simulink model "PID_PD_LQR_Control_Quadrotor"  (R2012b)
settings: Solver=ode3  StartTime=0.0  StopTime=105  FixedStep=0.01  RelTol=1e-2
libraries: vrlib x2
settings Model: Creator=hellb  LastModifiedBy=hellb
settings OptimizationCC: ExpressionDepthLimit=128
settings DebuggingCC: UnderspecifiedInitializationDetection=Simplified  MergeDetectMultiDrivingBlocksExec=error  SolverPrmCheckMsg=none  FrameProcessingCompatibilityMsg=error  StateNameClashWarn=none
settings CodeAppCC: CustomSymbolStrType=$N$R$M_T
settings GRTTargetCC: CodeReplacementLibrary=C89/C90 (ANSI)

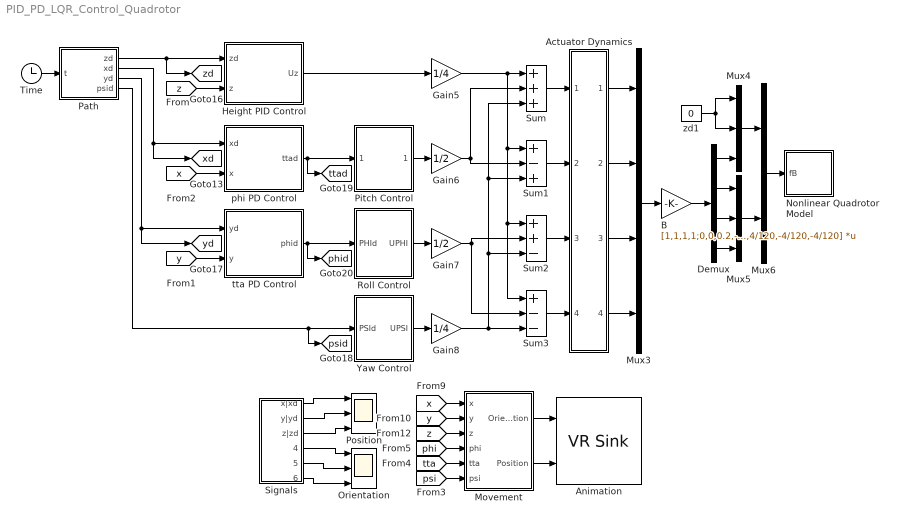
== system PID_PD_LQR_Control_Quadrotor ==
  Actuator Dynamics : Subsystem
  Animation : vrlib/VR Sink  InstantiateOnLoad=on  SampleTime=0.01  ViewEnable=on  RemoteChange=off  RemoteView=off  FieldsWritten=Drone.rotation.4.1.1.double#Drone.translation.3.1.1.double  WorldFileName=Animation\hummingbird.wrl  AutoView=off  VideoDimensions=[]  AllowVariableSize=off
  B : Gain  Gain=[1,1,1,1;0,0,0.2,-0.2;0.2,-0.2,0,0;4/120,4/120,-4/120,-4/120]  Multiplication=Matrix(K*u)
  Demux : Demux
  Gain5 : Gain  Gain=1/4
  Gain6 : Gain  Gain=1/2
  Gain7 : Gain  Gain=1/2
  Gain8 : Gain  Gain=1/4
  Height PID Control : Subsystem
  Movement : Subsystem
  Mux3 : Mux
  Mux4 : Mux  Inputs=3
  Mux5 : Mux  Inputs=3
  Mux6 : Mux  Inputs=2
  Nonlinear Quadrotor Model : Subsystem
  Orientation : Scope  NumInputPorts=3
      settings: YMin=-0.0225~-0.0075~-0.00015  YMax=0.0075~0.0225~0.00015  SaveName=Orientation
  Path : MATLAB Function  TreatAsAtomicUnit=on
      settings: PermitHierarchicalResolution=ParametersOnly
  Pitch Control : Subsystem
  Position : Scope  NumInputPorts=3
      settings: YMin=-0.25~-0.1~-0.25  YMax=3.25~1.3~3  SaveName=Position
  Roll Control : Subsystem
  Signals : Subsystem
  Sum : Sum  Inputs=+++
  Sum1 : Sum  Inputs=+-+
  Sum2 : Sum  Inputs=++-
  Sum3 : Sum  Inputs=+--
  Time : Clock
  Yaw Control : Subsystem
  phi PD Control : Subsystem
  tta PD Control : Subsystem
  zd1 : Constant  Value=0
  tag scope: phid=global, psid=global, ttad=global, xd=global, yd=global, zd=global
  wires:
  tta PD Control/1(phid) -> Roll Control/1(PHId), [phid]
  phi PD Control/1(ttad) -> Pitch Control/1(TTAd), [ttad]
  Height PID Control/1(Uz) -> Gain5/1
  Yaw Control/1(UPSI) -> Gain8/1
  Mux3/1 -> B/1
  B/1 -> Demux/1
  Demux/1 -> Mux4/3
  zd1/1 -> Mux4/1, Mux4/2
  Demux/2 -> Mux5/1
  Demux/3 -> Mux5/2
  Demux/4 -> Mux5/3
  Mux4/1 -> Mux6/1
  Mux5/1 -> Mux6/2
  [x] -> phi PD Control/2(x)
  Roll Control/1(UPHI) -> Gain7/1
  Pitch Control/1(UTTA) -> Gain6/1
  Gain5/1 -> Sum/1, Sum1/1, Sum3/1, Sum2/1
  [y] -> tta PD Control/2(y)
  Gain6/1 -> Sum1/2, Sum/2
  Gain7/1 -> Sum2/2, Sum3/2
  Gain8/1 -> Sum3/3, Sum2/3, Sum/3, Sum1/3
  [z] -> Height PID Control/2(z)
  Sum/1 -> Actuator Dynamics/1(U1)
  Sum1/1 -> Actuator Dynamics/2(U2)
  Sum2/1 -> Actuator Dynamics/3(U3)
  Sum3/1 -> Actuator Dynamics/4(U4)
  Actuator Dynamics/1(F1) -> Mux3/1
  Actuator Dynamics/2(F2) -> Mux3/2
  Actuator Dynamics/3(F3) -> Mux3/3
  Actuator Dynamics/4(F4) -> Mux3/4
  Mux6/1 -> Nonlinear Quadrotor Model/1(fB)
  Signals/1(x|xd) -> Position/1
  Signals/2(y|yd) -> Position/2
  Signals/3(z|zd) -> Position/3
  Signals/4(phi|phid) -> Orientation/1
  Signals/5(tta|ttad) -> Orientation/2
  Signals/6(psi|psid) -> Orientation/3
  Time/1 -> Path/1(t)
  Path/1(zd) -> [zd], Height PID Control/1(zd)
  Path/2(xd) -> phi PD Control/1(xd), [xd]
  Path/3(yd) -> tta PD Control/1(yd), [yd]
  Path/4(psid) -> Yaw Control/1(PSId), [psid]
  [phi] -> Movement/4(phi)
  [psi] -> Movement/6(psi)
  [tta] -> Movement/5(tta)
  [x] -> Movement/1(x)
  [z] -> Movement/3(z)
  [y] -> Movement/2(y)
  Movement/1(Orientation) -> Animation/1
  Movement/2(Position) -> Animation/2

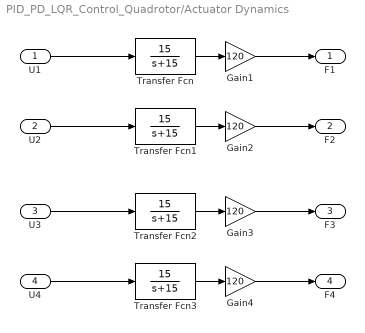
== system PID_PD_LQR_Control_Quadrotor/Actuator Dynamics ==
  U1 : Inport
  U2 : Inport  Port=2
  U3 : Inport  Port=3
  U4 : Inport  Port=4
  Gain{1..4} (4 alike) : Gain  Gain=120
  Transfer Fcn{,1..3} (4 alike) : TransferFcn  Numerator=[15]  Denominator=[1 15]
  F1 : Outport
  F2 : Outport  Port=2
  F3 : Outport  Port=3
  F4 : Outport  Port=4
  wires:
  Transfer Fcn1/1 -> Gain2/1
  U1/1 -> Transfer Fcn/1
  Gain2/1 -> F2/1
  Gain1/1 -> F1/1
  Transfer Fcn/1 -> Gain1/1
  Gain3/1 -> F3/1
  U3/1 -> Transfer Fcn2/1
  U4/1 -> Transfer Fcn3/1
  Transfer Fcn3/1 -> Gain4/1
  Gain4/1 -> F4/1
  U2/1 -> Transfer Fcn1/1
  Transfer Fcn2/1 -> Gain3/1

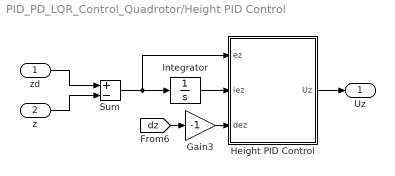
== system PID_PD_LQR_Control_Quadrotor/Height PID Control ==
  zd : Inport
  z : Inport  Port=2
  Gain3 : Gain  Gain=-1
  Height PID Control : MATLAB Function  TreatAsAtomicUnit=on
      settings: PermitHierarchicalResolution=ParametersOnly
  Integrator : Integrator
  Sum : Sum  Inputs=+-
  Uz : Outport
  wires:
  zd/1 -> Sum/1
  z/1 -> Sum/2
  Sum/1 -> Height PID Control/1(ez), Integrator/1
  Integrator/1 -> Height PID Control/2(iez)
  Gain3/1 -> Height PID Control/3(dez)
  [dz] -> Gain3/1
  Height PID Control/1(Uz) -> Uz/1

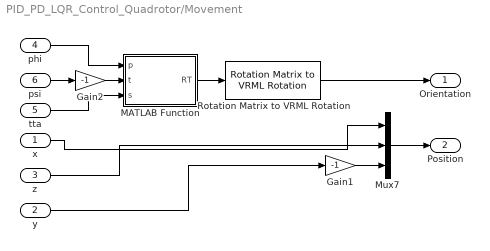
== system PID_PD_LQR_Control_Quadrotor/Movement ==
  x : Inport
  y : Inport  Port=2
  z : Inport  Port=3
  phi : Inport  Port=4
  tta : Inport  Port=5
  psi : Inport  Port=6
  Gain1 : Gain  Gain=-1
  Gain2 : Gain  Gain=-1
  MATLAB Function : MATLAB Function  TreatAsAtomicUnit=on
      settings: PermitHierarchicalResolution=ParametersOnly
  Mux7 : Mux  Inputs=3
  Rotation Matrix to VRML Rotation : vrlib/Utilities/Rotation Matrix to VRML Rotation  maxzero=1e-12
  Orientation : Outport
  Position : Outport  Port=2
  wires:
  Gain1/1 -> Mux7/3
  Rotation Matrix to VRML Rotation/1 -> Orientation/1
  Mux7/1 -> Position/1
  x/1 -> Mux7/1
  psi/1 -> Gain2/1
  MATLAB Function/1(RT) -> Rotation Matrix to VRML Rotation/1
  phi/1 -> MATLAB Function/1(p)
  y/1 -> Gain1/1
  Gain2/1 -> MATLAB Function/2(t)
  z/1 -> Mux7/2
  tta/1 -> MATLAB Function/3(s)

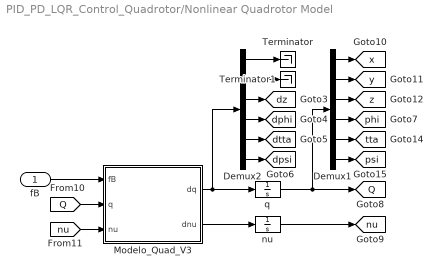
== system PID_PD_LQR_Control_Quadrotor/Nonlinear Quadrotor Model ==
  fB : Inport
  Demux1 : Demux  Outputs=6
  Demux2 : Demux  Outputs=6
  Modelo_Quad_V3 : MATLAB Function  TreatAsAtomicUnit=on
      settings: PermitHierarchicalResolution=ParametersOnly
  Terminator : Terminator
  Terminator1 : Terminator
  nu : Integrator  InitialCondition=[0,0,0,0,0,0]
  q : Integrator  InitialCondition=[0,0,0,0,0,0]
  tag scope: Q=global, dphi=global, dpsi=global, dtta=global, dz=global, nu=global, phi=global, psi=global, tta=global, x=global, y=global, z=global
  wires:
  Demux1/1 -> [x]
  Demux1/2 -> [y]
  Demux1/3 -> [z]
  Demux1/4 -> [phi]
  Demux2/3 -> [dz]
  Modelo_Quad_V3/1(dq) -> Demux2/1, q/1
  Demux2/6 -> [dpsi]
  Demux2/4 -> [dphi]
  nu/1 -> [nu]
  [nu] -> Modelo_Quad_V3/3(nu)
  Demux2/5 -> [dtta]
  Demux1/6 -> [psi]
  [Q] -> Modelo_Quad_V3/2(q)
  q/1 -> Demux1/1, [Q]
  Modelo_Quad_V3/2(dnu) -> nu/1
  fB/1 -> Modelo_Quad_V3/1(fB)
  Demux1/5 -> [tta]
  Demux2/1 -> Terminator/1
  Demux2/2 -> Terminator1/1

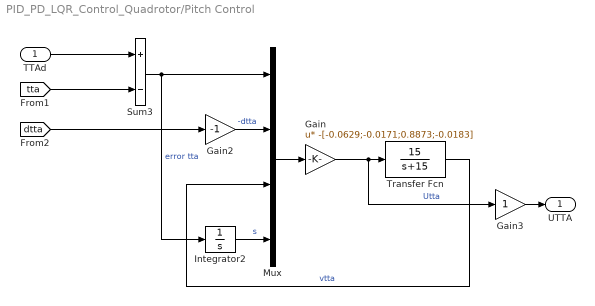
== system PID_PD_LQR_Control_Quadrotor/Pitch Control ==
  TTAd : Inport
  Gain : Gain  Gain=-[-0.0629;-0.0171;0.8873;-0.0183]  Multiplication=Matrix(u*K)
  Gain2 : Gain  Gain=-1
  Gain3 : Gain
  Integrator2 : Integrator
  Mux : Mux
  Sum3 : Sum  Inputs=+-
  Transfer Fcn : TransferFcn  Numerator=[15]  Denominator=[1 15]
  UTTA : Outport
  wires:
  Gain/1 -> Gain3/1, Transfer Fcn/1  "Utta"
  Transfer Fcn/1 -> Mux/3  "vtta"
  Sum3/1 -> Integrator2/1, Mux/1  "error tta"
  TTAd/1 -> Sum3/1
  Gain2/1 -> Mux/2  "-dtta"
  Mux/1 -> Gain/1
  Integrator2/1 -> Mux/4  "s"
  [tta] -> Sum3/2
  [dtta] -> Gain2/1
  Gain3/1 -> UTTA/1

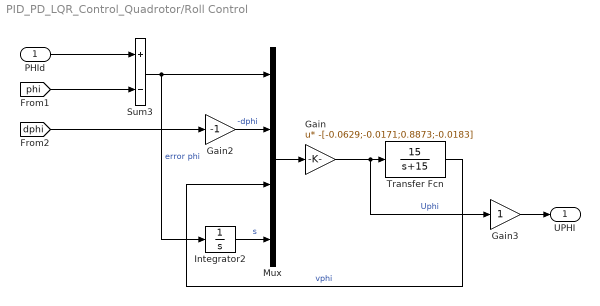
== system PID_PD_LQR_Control_Quadrotor/Roll Control ==
  PHId : Inport
  Gain : Gain  Gain=-[-0.0629;-0.0171;0.8873;-0.0183]  Multiplication=Matrix(u*K)
  Gain2 : Gain  Gain=-1
  Gain3 : Gain
  Integrator2 : Integrator
  Mux : Mux
  Sum3 : Sum  Inputs=+-
  Transfer Fcn : TransferFcn  Numerator=[15]  Denominator=[1 15]
  UPHI : Outport
  wires:
  Gain/1 -> Gain3/1, Transfer Fcn/1  "Uphi"
  Transfer Fcn/1 -> Mux/3  "vphi"
  Sum3/1 -> Integrator2/1, Mux/1  "error phi"
  PHId/1 -> Sum3/1
  Gain2/1 -> Mux/2  "-dphi"
  Mux/1 -> Gain/1
  Integrator2/1 -> Mux/4  "s"
  [phi] -> Sum3/2
  [dphi] -> Gain2/1
  Gain3/1 -> UPHI/1

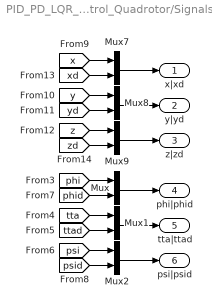
== system PID_PD_LQR_Control_Quadrotor/Signals ==
  Mux{,1..2,7..9} (6 alike) : Mux  Inputs=2
  x|xd : Outport
  y|yd : Outport  Port=2
  z|zd : Outport  Port=3
  phi|phid : Outport  Port=4
  tta|ttad : Outport  Port=5
  psi|psid : Outport  Port=6
  wires:
  Mux/1 -> phi|phid/1
  Mux2/1 -> psi|psid/1
  [psi] -> Mux2/1
  [psid] -> Mux2/2
  [tta] -> Mux1/1
  [ttad] -> Mux1/2
  Mux1/1 -> tta|ttad/1
  [phid] -> Mux/2
  [yd] -> Mux8/2
  [y] -> Mux8/1
  Mux7/1 -> x|xd/1
  [xd] -> Mux7/2
  [z] -> Mux9/1
  Mux9/1 -> z|zd/1
  [zd] -> Mux9/2
  [x] -> Mux7/1
  Mux8/1 -> y|yd/1
  [phi] -> Mux/1

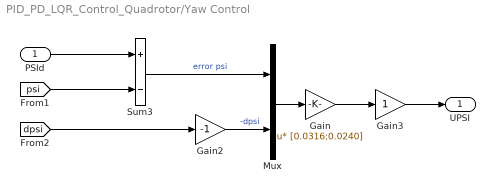
== system PID_PD_LQR_Control_Quadrotor/Yaw Control ==
  PSId : Inport
  Gain : Gain  Gain=[0.0316;0.0240]  Multiplication=Matrix(u*K)
  Gain2 : Gain  Gain=-1
  Gain3 : Gain
  Mux : Mux  Inputs=2
  Sum3 : Sum  Inputs=+-
  UPSI : Outport
  wires:
  Gain/1 -> Gain3/1
  Sum3/1 -> Mux/1  "error psi"
  PSId/1 -> Sum3/1
  Gain2/1 -> Mux/2  "-dpsi"
  Mux/1 -> Gain/1
  [psi] -> Sum3/2
  [dpsi] -> Gain2/1
  Gain3/1 -> UPSI/1

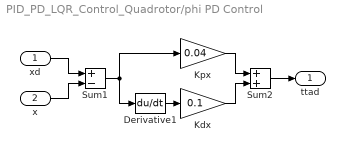
== system PID_PD_LQR_Control_Quadrotor/phi PD Control ==
  xd : Inport
  x : Inport  Port=2
  Derivative1 : Derivative
  Kdx : Gain  Gain=0.1
  Kpx : Gain  Gain=0.04
  Sum1 : Sum  Inputs=+-
  Sum2 : Sum
  ttad : Outport
  wires:
  Sum1/1 -> Kpx/1, Derivative1/1
  Sum2/1 -> ttad/1
  Derivative1/1 -> Kdx/1
  Kpx/1 -> Sum2/1
  Kdx/1 -> Sum2/2
  xd/1 -> Sum1/1
  x/1 -> Sum1/2

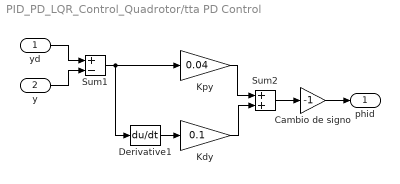
== system PID_PD_LQR_Control_Quadrotor/tta PD Control ==
  yd : Inport
  y : Inport  Port=2
  Cambio de signo : Gain  Gain=-1
  Derivative1 : Derivative
  Kdy : Gain  Gain=0.1
  Kpy : Gain  Gain=0.04
  Sum1 : Sum  Inputs=+-
  Sum2 : Sum
  phid : Outport
  wires:
  Sum1/1 -> Derivative1/1, Kpy/1
  Cambio de signo/1 -> phid/1
  Derivative1/1 -> Kdy/1
  Kpy/1 -> Sum2/1
  Kdy/1 -> Sum2/2
  Sum2/1 -> Cambio de signo/1
  yd/1 -> Sum1/1
  y/1 -> Sum1/2

== matlab function PID_PD_LQR_Control_Quadrotor/Height PID Control/Height PID Control ==
  data: ez input; Uz output; iez input; dez input
function Uz = fcn(ez,iez,dez)

% kpz = 0.1242;
% kiz = 0.042;
% kdz = 0.1565;

kpz = 0.33;
kiz = 0.15;
kdz = 0.25;

Uz = kpz*ez + kiz*iez + kdz*dez;

== matlab function PID_PD_LQR_Control_Quadrotor/Movement/MATLAB Function ==
  data: p input; RT output; t input; s input
function RT = fcn(p,t,s)

RT = [cos(t)*cos(s);
    sin(t)*cos(s)*sin(p)-sin(s)*cos(p);
    sin(t)*cos(s)*cos(p)+sin(s)*sin(p);
    cos(t)*sin(s);
    sin(t)*sin(s)*sin(p)+cos(s)*cos(p);
    sin(t)*sin(s)*cos(p)-cos(s)*sin(p);
    -sin(t);
    cos(t)*sin(p);
    cos(t)*cos(p)];

== matlab function PID_PD_LQR_Control_Quadrotor/Path ==
  data: t input; zd output; xd output; yd output; psid output
function [zd,xd,yd,psid] = fcn(t)

    zd = 0;
    xd = 0;
    yd = 0;
    psid = 0;

if (t<15)
    zd = 0.5;
    xd = 0.2;
    yd = 0.6;
    psid = 0.1;
elseif (t>=15 && t<30)
    zd = 1;
    xd = 1;
    yd = 1;
    psid = 0.5;
elseif (t>=30 && t<45)
    zd = 2.5;
    xd = 2;
    yd = 0.3;
    psid = 0;
elseif (t>=45 && t<60)
    zd = 0.7;
    xd = 3;
    yd = 1.2;
    psid = 0;
elseif (t>=60 && t<75)
    zd = 3;
    xd = -0.5;
    yd = -1;
    psid = -0.25;
elseif (t>=75 && t<90)
    zd = 1;
    xd = -1.5;
    yd = -2.25;
    psid = 0.25;
elseif (t>=90 && t<105)
    zd = 0.5;
    xd = 0;
    yd = 0;
    psid = 0;
end

== matlab function PID_PD_LQR_Control_Quadrotor/Nonlinear Quadrotor Model/Modelo_Quad_V3 ==
  data: dq output; fB input; dnu output; q input; nu input
function [dq,dnu] = fcn(fB,q,nu)

g = 9.81;
m = 1.4;
%l = 0.2;
Ix = 0.03;
Iy = 0.03;
Iz = 0.03;
%kd = 0.05;
r = [0.0;0.0;0.0];

phi = q(4,1);
tta = q(5,1);
psi = q(6,1);

sp = sin(phi);
cp = cos(phi);
% tp = tan(phi);

st = sin(tta);
ct = cos(tta);
tt = tan(tta);

ss = sin(psi);
cs = cos(psi);
% ts = tan(psi);

R = [ct*cs  st*cs*sp-ss*cp  st*cs*cp+ss*sp;
     ct*ss  st*ss*sp+cs*cp  st*ss*cp-cs*sp;
      -st       ct*sp          ct*cp     ];

W = [1 sp*tt  cp*tt;
     0   cp    -sp;
     0 sp/ct  cp/ct];

J = [R(1,1) R(1,2) R(1,3)   0      0      0;
     R(2,1) R(2,2) R(2,3)   0      0      0;
     R(3,1) R(3,2) R(3,3)   0      0      0;
       0      0      0    W(1,1) W(1,2) W(1,3);
       0      0      0    W(2,1) W(2,2) W(2,3);
       0      0      0    W(3,1) W(3,2) W(3,3)];
   
w = [nu(4,1);nu(5,1);nu(6,1)];
   
Sw = [   0    -w(3,1)  w(2,1);
       w(3,1)    0    -w(1,1);
      -w(2,1)  w(1,1)    0  ];

Sr = [   0    -r(3,1)  r(2,1);
       r(3,1)    0    -r(1,1);
      -r(2,1)  r(1,1)    0  ];

ez = [0; 0; 1];

gB11 = m*g*(R')*ez;
gB21 = m*g*Sr*(R')*ez;

gB = [gB11(1,1);
      gB11(2,1);
      gB11(3,1);
      gB21(1,1);
      gB21(2,1);
      gB21(3,1)];

I = [Ix 0 0; 0 Iy 0; 0 0 Iz];
  
CB11 = m*Sw;
CB12 = -(m*Sr*Sw)';
CB21 = m*Sr*Sw;
CB22 = Sw*I;

CB = [CB11(1,1) CB11(1,2) CB11(1,3) CB12(1,1) CB12(1,2) CB12(1,3);
      CB11(2,1) CB11(2,2) CB11(2,3) CB12(2,1) CB12(2,2) CB12(2,3);
      CB11(3,1) CB11(3,2) CB11(3,3) CB12(3,1) CB12(3,2) CB12(3,3);
      CB21(1,1) CB21(1,2) CB21(1,3) CB22(1,1) CB22(1,2) CB22(1,3);
      CB21(2,1) CB21(2,2) CB21(2,3) CB22(2,1) CB22(2,2) CB22(2,3);
      CB21(3,1) CB21(3,2) CB21(3,3) CB22(3,1) CB22(3,2) CB22(3,3)];
  
MB11 = m*eye(3);
MB12 = -m*Sr;
MB21 = m*Sr;

MB = [MB11(1,1) MB11(1,2) MB11(1,3) MB12(1,1) MB12(1,2) MB12(1,3);
      MB11(2,1) MB11(2,2) MB11(2,3) MB12(2,1) MB12(2,2) MB12(2,3);
      MB11(3,1) MB11(3,2) MB11(3,3) MB12(3,1) MB12(3,2) MB12(3,3);
      MB21(1,1) MB21(1,2) MB21(1,3)  I(1,1)    I(1,2)    I(1,3)  ;
      MB21(2,1) MB21(2,2) MB21(2,3)  I(2,1)    I(2,2)    I(2,3)  ;
      MB21(3,1) MB21(3,2) MB21(3,3)  I(3,1)    I(3,2)    I(3,3) ];
  
fB = [fB(1);
      fB(2);
      fB(3);
      fB(4);
      fB(5);
      fB(6)];

dnu = MB\(fB-CB*nu-gB);
dq = J*nu;
